simulink model "step1"  (R2021b)
settings: Solver=VariableStepAuto  StartTime=0.0  StopTime=10.0  RelTol=1e-3
settings Model: Creator=just cookie file  LastModifiedBy=just cookie file

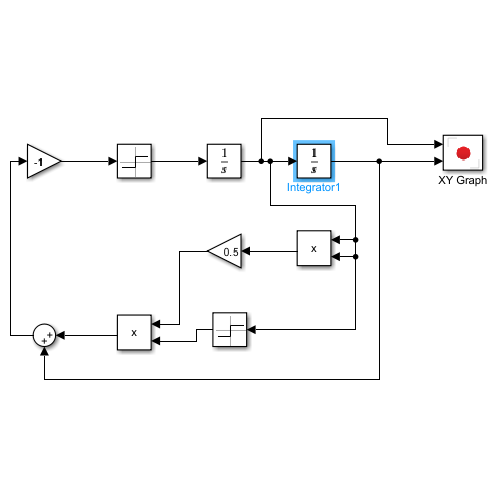
[thumbnail: Simulink's stored preview of the top-level diagram]
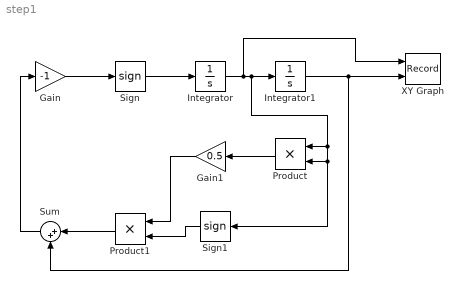
== system step1 ==
  Gain : Gain  Gain=-1
  Gain1 : Gain  Gain=0.5
  Integrator : Integrator  InitialCondition=1
  Integrator1 : Integrator
  Product : Product
  Product1 : Product
  Sign : Signum  ZeroCross=off
  Sign1 : Signum  ZeroCross=off
  Sum : Sum  Inputs=|++
  XY Graph : Record  FileSettingsInternal="{\"entries\":[{\"content\":{\"excelSettings\":{\"content\":{},\"type\":\"Streamout.ExcelSettings\"}},\"type\":\"Streamout.FileSettingStorage\",\"uuid\":\"c8f97f76-8aca-4c8a-98d0-985f608419e3\"}],\"packageUris\":[\"http://schema.mathworks.com/mf0/streamout_blocks/R2020a\"],\"version\":\"1.0\"}"  Layout=[1 1]  SignalsInternal="{\"entries\":[{\"content\":{\"signals\":[{\"content\":{\"blockPath\":[\"untitled/XY Graph\"],\"channel\":[],\"dimensions\":[1],\"domain\":\"untitled/XY Graph\",\"lineColor\":\"#a2142f\",\"plots\":[1],\"port\":1,\"sid\":[\"\"],\"signalID\":245,\"signalName\":\"Integrator\"},\"type\":\"RecordBlkView.Signal\",\"uuid\":\"4b73d92a-c5ee-4c1c-bdc2-76d8caa480e5\"},{\"content\":{\"blockPath\":[\"untitled/XY Graph\"],\"channel\":[],\"dimensions\":[1],\"domain\":\"untitled/XY Graph\",\"lineColor\":\"#139fff\",\"plots\":[1],\"port\":2,\"sid\":[\"\"],\"signalID\":249,\"signalName\":\"Transfer Fcn\"},\"type\":\"RecordBlkView.Signal\",\"uuid\":\"a0303583-cb2e-4d58-a411-69bb5ca0389a\"}]},\"type\":\"RecordBlkView.InputSignals\",\"uuid\":\"27bc7320-6a68-46b5-8cdf-2f48da4e8aec\"}],\"packageUris\":[\"http://schema.mathworks.com/mf0/streamout_blocks/R2020a\"],\"version\":\"1.0\"}"  VisualizationBindings="{\"xyplotplugin\":{\"info\":[{\"series\":[{\"bindingParametersList\":[{\"parameter\":\"X-Axis\",\"signalID\":245,\"signalName\":\"Integrator\"},{\"parameter\":\"Y-Axis\",\"signalID\":249,\"signalName\":\"Transfer Fcn\"}],\"seriesID\":39876}],\"subplotID\":1}]}}"  CompatibilityTag=XY
  wires:
  Sum/1 -> Gain/1
  Gain/1 -> Sign/1
  Sign/1 -> Integrator/1
  Integrator/1 -> Product/2, Sign1/1, Product/1, Integrator1/1, XY Graph/1
  Integrator1/1 -> Sum/2, XY Graph/2
  Product/1 -> Gain1/1
  Product1/1 -> Sum/1
  Sign1/1 -> Product1/2
  Gain1/1 -> Product1/1
